simulink model "Simulation_DC_ObsEstParams"  (R2021a)
settings: Solver=ode5  StartTime=ti  StopTime=tf  FixedStep=Ts/40  RelTol=1e-3
undefined symbols (not defined in the file): A_real, B_real, Cx_real, Dx_real, f, IC, Noise, torque, u0, umax
libraries: simulink x1
settings Model: Creator=perruquetti  LastModifiedBy=perruquetti
settings SolverCC: AlgebraicLoopSolver=TrustRegion
settings DataIOCC: ReturnWorkspaceOutputs=off
settings DebuggingCC: SFMachineParentedDataDiag=warning  ArithmeticOperatorsInVariantConditions=warning
settings SFSimCC: SimUseLocalCustomCode=off  CustomCodeUndefinedFunction=UseInterfaceOnly
settings RTWCC: RTWUseLocalCustomCode=off

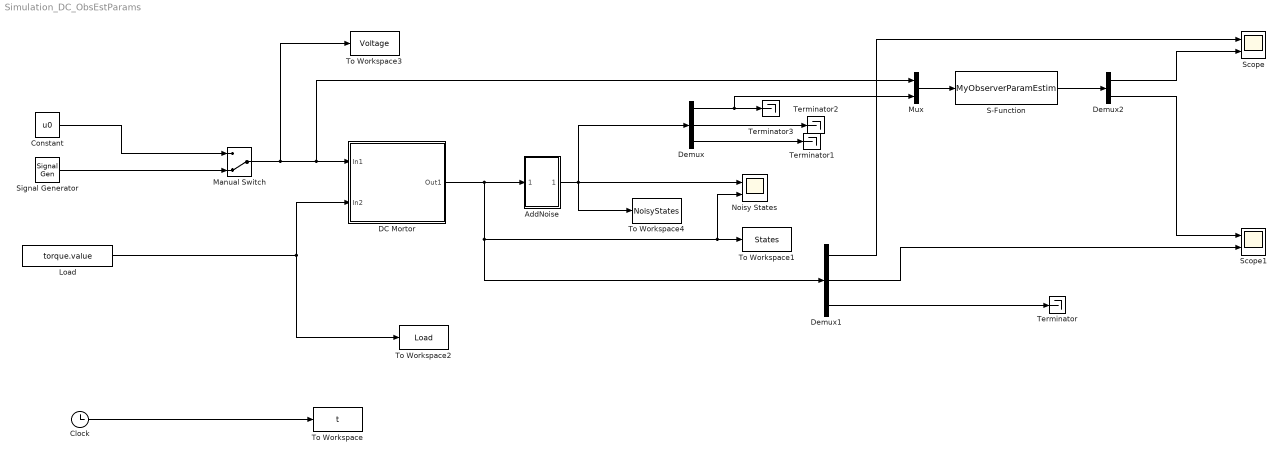
== system Simulation_DC_ObsEstParams ==
  AddNoise : Subsystem
  Clock : Clock
  Constant : Constant  Value=u0
  DC Mortor : Subsystem
      mask Display: image('motor2.png');
  Demux : Demux  Outputs=3
  Demux1 : Demux  Outputs=3
  Demux2 : Demux  Outputs=2
  Load : Constant  Value=torque.value
  Manual Switch : ManualSwitch  CurrentSetting=0
  Mux : Mux  Inputs=2
  Noisy States : Scope  NumInputPorts=2
  S-Function : S-Function  FunctionName=MyObserverParamEstim  SFunctionDeploymentMode=off  EnableBusSupport=off
  Scope : Scope  NumInputPorts=2
  Scope1 : Scope  NumInputPorts=2
  Signal Generator : SignalGenerator  Amplitude=u0  Frequency=f  Units=rad/sec
  Terminator{,1..3} (4 alike) : Terminator
  To Workspace : ToWorkspace  VariableName=t  SampleTime=-1
  To Workspace1 : ToWorkspace  VariableName=States  SampleTime=-1
  To Workspace2 : ToWorkspace  VariableName=Load  SampleTime=-1
  To Workspace3 : ToWorkspace  VariableName=Voltage  SampleTime=-1
  To Workspace4 : ToWorkspace  VariableName=NoisyStates  SampleTime=-1
  wires:
  Clock/1 -> To Workspace/1
  DC Mortor/1(Out1) -> AddNoise/1(In1), Demux1/1, Noisy States/2, To Workspace1/1
  Load/1 -> DC Mortor/2(In2), To Workspace2/1
  Constant/1 -> Manual Switch/1
  Signal Generator/1 -> Manual Switch/2
  Manual Switch/1 -> To Workspace3/1, Mux/1, DC Mortor/1(In1)
  AddNoise/1(Out1) -> Demux/1, To Workspace4/1, Noisy States/1
  S-Function/1 -> Demux2/1
  Demux1/1 -> Scope/1
  Demux1/2 -> Scope1/2
  Demux2/2 -> Scope1/1
  Demux1/3 -> Terminator/1
  Demux2/1 -> Scope/2
  Mux/1 -> S-Function/1
  Demux/3 -> Terminator1/1
  Demux/2 -> Terminator2/1
  Demux/1 -> Mux/2, Terminator3/1

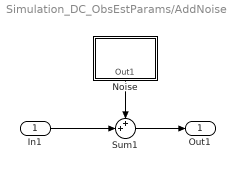
== system Simulation_DC_ObsEstParams/AddNoise ==
  In1 : Inport
  Noise : Subsystem
  Sum1 : Sum  Inputs=++|
  Out1 : Outport
  wires:
  In1/1 -> Sum1/2
  Sum1/1 -> Out1/1
  Noise/1(Out1) -> Sum1/1

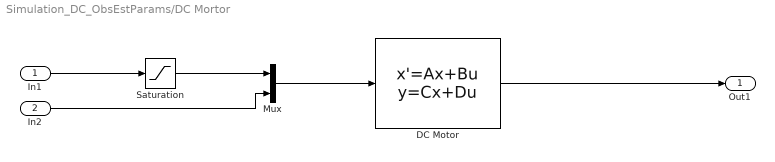
== system Simulation_DC_ObsEstParams/DC Mortor ==
  In1 : Inport
  In2 : Inport  Port=2
  DC Motor : StateSpace  A=A_real  B=B_real  C=Cx_real  D=Dx_real  InitialCondition=IC.state
  Mux : Mux  Inputs=2
  Saturation : Saturate  UpperLimit=umax  LowerLimit=-umax
  Out1 : Outport  VectorParamsAs1DForOutWhenUnconnected=off
  wires:
  DC Motor/1 -> Out1/1
  In1/1 -> Saturation/1
  Saturation/1 -> Mux/1
  Mux/1 -> DC Motor/1
  In2/1 -> Mux/2

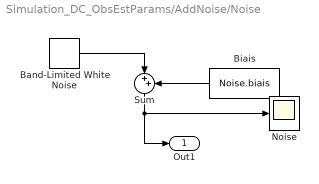
== system Simulation_DC_ObsEstParams/AddNoise/Noise ==
  Band-Limited White Noise : simulink/Sources/Band-Limited White Noise  Cov=Noise.power  Ts=Noise.sampling  seed=Noise.seed
  Biais : Constant  Value=Noise.biais
  Noise : Scope
  Sum : Sum  Inputs=|++
  Out1 : Outport
  wires:
  Sum/1 -> Out1/1, Noise/1
  Biais/1 -> Sum/2
  Band-Limited White Noise/1 -> Sum/1
